simulink model "slexVariantControlPorts_org"  (Simulink 10.0)
settings: Solver=FixedStepAuto  StartTime=0.0  StopTime=10.0  RelTol=1e-3  EnableMultiTasking=on
PreLoadFcn:
  | addpath(fileparts(which(bdroot)));
PostLoadFcn:
  | V = Simulink.Parameter(int32(1));
  | V.StorageClass = 'Define (Custom)';
  | V.CoderInfo.CustomAttributes.HeaderFile='variant_defines.h';
settings Model: Creator=The MathWorks, Inc.  LastModifiedBy=bhisma
settings DataIOCC: LimitDataPoints=on  ReturnWorkspaceOutputs=on  OutputSaveName=out1
settings OptimizationCC: LifeSpan=1  EfficientTunableParamExpr=on
settings DebuggingCC: UnderspecifiedInitializationDetection=Simplified  MergeDetectMultiDrivingBlocksExec=error  AllowSymbolicDim=off  PregeneratedLibrarySubsystemCodeDiagnostic=none
settings SFSimCC: MATLABDynamicMemAlloc=off
settings RTWCC: Description=Embedded Coder  SystemTargetFile=ert.tlc  TemplateMakefile=ert_default_tmf  GenerateReport=on  IncludeHyperlinkInReport=on  LaunchReport=on
settings CodeAppCC: IgnoreCustomStorageClasses=off  MaxIdLength=127  CustomSymbolStrModelFcn=$N
settings ERTTargetCC: MultiwordLength=2048  GenerateSampleERTMain=on  ERTCustomFileTemplate=example_file_process.tlc  ConvertIfToSwitch=off  SuppressUnreachableDefaultCases=off
settings ConfigComp: CovExternalEMLEnable=off

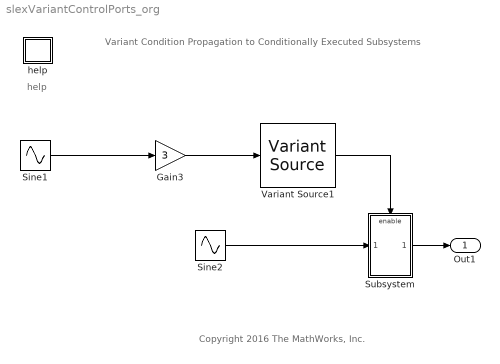
== system slexVariantControlPorts_org ==
  note: Variant Condition Propagation to Conditionally Executed Subsystems
  note: Copyright 2016 The MathWorks, Inc.
  note: help
  Gain3 : Gain  Gain=3
  Sine1 : Sin  SineType=Sample based  SampleTime=0.2
  Sine2 : Sin  SineType=Sample based  Amplitude=2  SampleTime=0.2
  Subsystem : Subsystem
  Variant Source1 : VariantSource  VariantControls=DataTag0  ShowConditionOnBlock=on
      settings: GeneratePreprocessorConditionals=on  AllowZeroVariantControls=on
  help : Subsystem
      mask Display: disp('?')
  Out1 : Outport  VectorParamsAs1DForOutWhenUnconnected=off
  wires:
  Sine1/1 -> Gain3/1
  Gain3/1 -> Variant Source1/1
  Subsystem/1(Out1) -> Out1/1
  Variant Source1/1 -> Subsystem/Enable
  Sine2/1 -> Subsystem/1(In1)

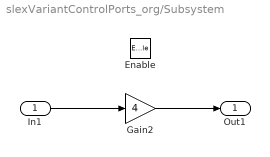
== system slexVariantControlPorts_org/Subsystem ==
  In1 : Inport
  Enable : EnablePort
  Gain2 : Gain  Gain=4
  Out1 : Outport  VectorParamsAs1DForOutWhenUnconnected=off
  wires:
  In1/1 -> Gain2/1
  Gain2/1 -> Out1/1

== system slexVariantControlPorts_org/help ==
  note: This illustrates the propagation of variant conditions to conditionally executed subsystems.
      |
      | When a control port (Enable, Trigger, Function-Call, Action) of a conditionally executed subsystem or Model block becomes conditional, the block is assigned the variant condition of the signal connected to the control port. The condition assigned to the subsystem or block is then propagated to blocks connected to its signal input and output ports. In this example, this means the Sine2 and Out1 will have the same variant condition as the Enabled Subsystem.
